simulink model "howard_lin_r2013a_20160128"  (R2013a)
settings: Solver=ode45  StartTime=0.0  StopTime=tFinal  RelTol=1e-3
PreLoadFcn:
  | OAT=30;
  | Temp=68;
  | 
  | Rn=29;
  | Rx=69;
  | Tn=180;
  | Tx=120;
  | 
  | Hc=114/86400;
  | Ha=1.61/86400;
  | %Hf=1.08/86400;
  | Hf=1.745/86400;
  | Ho=283/86400;
  | 
  | tau=40;
  | FILTER_DELAY = 5;
  | 
  | K2=1;
  | K3=1;
  | Ki=1e-5;
  | Kp=2;
  | Kd=800;
  | Kf=1;
  | compGain=400;  % gain in TCOMP of house control
  | Kei=Ki*2;
  | Kep=Kp*2;
  | 
  | % From match to thermo20160128.xlsx
  | sNoise=0.001;
  | SET = [0 60 18861 18862; 68 62 68 68]';
  | otherHeat=[0 1000 6000; .0002 .001 .0005]';
  | tFinal = 24132;
InitFcn:
  | Ta0=Temp;
  | Tw0 = (Temp*Ha + OAT*Ho)/(Ho+Ha);
  | Tb0=max(min(interp1([Rn Rx],[Tn Tx],OAT), Tn),Tx);
  | Tc0 = ((Ha+Hc)*Ta0 - Ha*Tw0) / Hc;
  | D0 =max(min( Hc*(Tc0-Ta0)/(Hf*(Tb0-Tc0)), 1), 1e-32);
settings Model: Creator=210023782  LastModifiedBy=210023782
settings DataIOCC: InitialState=xinHouse  LimitDataPoints=off  SaveState=on  StateSaveName=xoutHouse

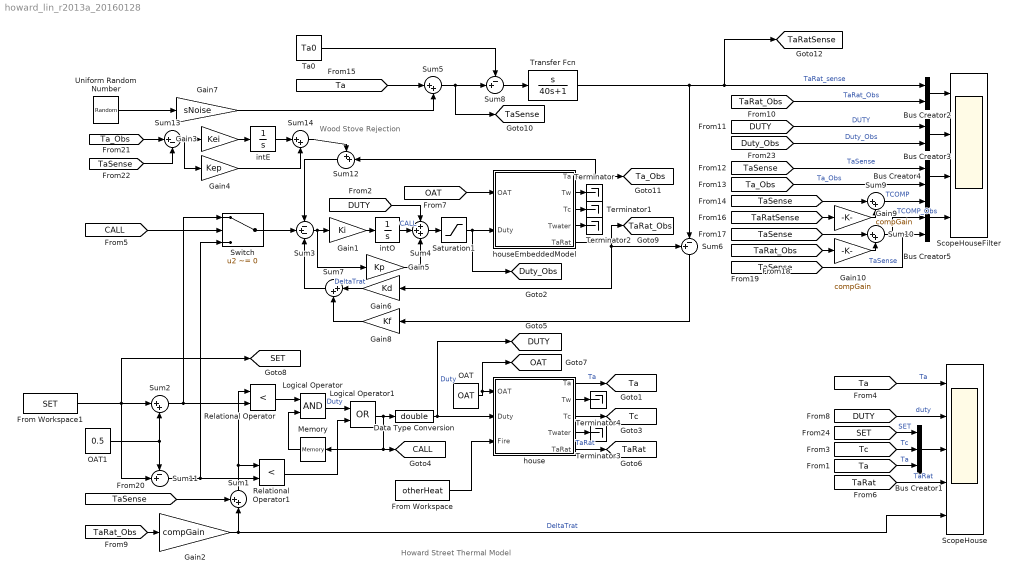
== system howard_lin_r2013a_20160128 ==
  note: Howard Street Thermal Model
  note: Wood Stove Rejection
  Bus Creator1 : BusCreator  Inputs=3
  Bus Creator2 : BusCreator  Inputs=2
  Bus Creator3 : BusCreator  Inputs=2
  Bus Creator4 : BusCreator  Inputs=2
  Bus Creator5 : BusCreator  Inputs=3
  Data Type Conversion : DataTypeConversion  OutDataTypeStr=double
  From Workspace : FromWorkspace  VariableName=otherHeat  SampleTime=1  OutputAfterFinalValue=Holding final value
  From Workspace1 : FromWorkspace  VariableName=SET  SampleTime=1  OutputAfterFinalValue=Holding final value
  Gain1 : Gain  Gain=Ki
  Gain10 : Gain  Gain=compGain
  Gain2 : Gain  Gain=compGain
  Gain3 : Gain  Gain=Kei
  Gain4 : Gain  Gain=Kep
  Gain5 : Gain  Gain=Kp
  Gain6 : Gain  Gain=Kd
  Gain7 : Gain  Gain=sNoise
  Gain8 : Gain  Gain=Kf
  Gain9 : Gain  Gain=compGain
  Logical Operator : Logic  AllPortsSameDT=off  OutDataTypeStr=boolean
  Logical Operator1 : Logic  Operator=OR  AllPortsSameDT=off  OutDataTypeStr=boolean
  Memory : Memory
  OAT : Constant  Value=OAT
  OAT1 : Constant  Value=0.5
  Relational Operator : RelationalOperator  Operator=<  OutDataTypeStr=boolean
  Relational Operator1 : RelationalOperator  Operator=<  OutDataTypeStr=boolean
  Saturation1 : Saturate  UpperLimit=1.0  LowerLimit=1e-32
  ScopeHouse : Scope  NumInputPorts=5
      settings: ShowLegends=on  YMin=-75~-40~-5~-5~-5  YMax=75~70~5~5~5  Decimation=2
  ScopeHouseFilter : Scope  NumInputPorts=4
      settings: ShowLegends=on  YMin=-75~-40~-10~-5  YMax=75~70~10~5  SaveName=ScopeData4  Decimation=2
  Sum1 : Sum  Inputs=++|
  Sum{2,5,7,9..10,14} (6 alike) : Sum  Inputs=|++
  Sum11 : Sum  Inputs=-+|
  Sum12 : Sum  Inputs=++|
  Sum13 : Sum  Inputs=|+-
  Sum3 : Sum  Inputs=-+-
  Sum4 : Sum  Inputs=+++
  Sum6 : Sum  Inputs=+-|
  Sum8 : Sum  Inputs=-+|
  Switch : Switch  Criteria=u2 ~= 0
  Ta0 : Constant  Value=Ta0
  Terminator{,1..4} (5 alike) : Terminator
  Transfer Fcn : TransferFcn  Numerator=[1 0]  Denominator=[40 1]
  Uniform Random Number : UniformRandomNumber  SampleTime=FILTER_DELAY
  house : Subsystem
  houseEmbeddedModel : Subsystem
  intE : Integrator  LimitOutput=on  UpperSaturationLimit=10  LowerSaturationLimit=-10
  intO : Integrator  LimitOutput=on  UpperSaturationLimit=1  LowerSaturationLimit=-1
  tag scope: CALL=global, DUTY=global, Duty_Obs=global, OAT=global, SET=global, Ta=global, TaRat=global, TaRatSense=global, TaRat_Obs=global, TaSense=global, Ta_Obs=global, Tc=global
  wires:
  OAT/1 -> [OAT], house/1(OAT)
  house/1(Ta) -> [Ta]  "Ta"
  house/2(Tw) -> Terminator4/1
  house/3(Tc) -> [Tc]
  house/4(Twater) -> Terminator3/1
  Bus Creator2/1 -> ScopeHouseFilter/1
  [Ta] -> ScopeHouse/1  "Ta"
  house/5(TaRat) -> [TaRat]  "TaRat"
  [TaRat] -> ScopeHouse/4  "TaRat"
  Logical Operator/1 -> Logical Operator1/1  "Duty"
  Gain2/1 -> ScopeHouse/5, Sum1/2  "DeltaTrat"
  [OAT] -> houseEmbeddedModel/1(OAT)
  houseEmbeddedModel/1(Ta) -> Sum12/2, [Ta_Obs]
  Sum3/1 -> Gain1/1, Gain5/1
  Sum4/1 -> Saturation1/1
  Gain1/1 -> intO/1
  Saturation1/1 -> houseEmbeddedModel/2(Duty), [Duty_Obs]
  [TaRat_Obs] -> Gain2/1
  houseEmbeddedModel/5(TaRat) -> Sum6/1, Gain6/1, [TaRat_Obs]
  houseEmbeddedModel/2(Tw) -> Terminator/1
  houseEmbeddedModel/3(Tc) -> Terminator1/1
  houseEmbeddedModel/4(Twater) -> Terminator2/1
  Uniform Random Number/1 -> Gain7/1
  Sum5/1 -> [TaSense], Sum8/2
  Transfer Fcn/1 -> [TaRatSense], Bus Creator2/1, Sum6/2  "TaRat_sense"
  Sum6/1 -> Gain8/1
  Sum7/1 -> Sum3/3
  Gain6/1 -> Sum7/1  "DeltaTrat"
  Gain8/1 -> Sum7/2
  [TaRat_Obs] -> Bus Creator2/2  "TaRat_Obs"
  [DUTY] -> Bus Creator3/1  "DUTY"
  Bus Creator3/1 -> ScopeHouseFilter/2
  [Ta] -> Sum5/1
  Gain7/1 -> Sum5/2
  Ta0/1 -> Sum8/1
  Sum8/1 -> Transfer Fcn/1
  [TaSense] -> Bus Creator4/1  "TaSense"
  [Ta_Obs] -> Bus Creator4/2  "Ta_Obs"
  Bus Creator4/1 -> ScopeHouseFilter/3
  Bus Creator5/1 -> ScopeHouseFilter/4
  [TaRatSense] -> Gain9/1
  [TaSense] -> Sum9/1
  Gain9/1 -> Sum9/2
  Sum9/1 -> Bus Creator5/1  "TCOMP"
  [TaRat_Obs] -> Gain10/1
  [TaSense] -> Sum10/1
  Gain10/1 -> Sum10/2
  Sum10/1 -> Bus Creator5/2  "TCOMP_Obs"
  [TaSense] -> Bus Creator5/3  "TaSense"
  Sum1/1 -> Relational Operator1/1, Relational Operator/1
  OAT1/1 -> Sum11/1, Sum2/2
  Sum2/1 -> Switch/1, Relational Operator/2
  Relational Operator/1 -> Logical Operator/1
  [TaSense] -> Sum1/1
  Data Type Conversion/1 -> house/2(Duty), [DUTY]  "Duty"
  Memory/1 -> Logical Operator/2
  Relational Operator1/1 -> Logical Operator1/2
  Sum11/1 -> Relational Operator1/2, Switch/3
  intO/1 -> Sum4/2  "CALL"
  Gain5/1 -> Sum4/3
  [DUTY] -> Sum4/1
  Switch/1 -> Sum3/2
  [CALL] -> Switch/2
  From Workspace/1 -> house/3(Fire)
  Sum12/1 -> Sum3/1
  [Ta_Obs] -> Sum13/1
  [TaSense] -> Sum13/2
  Sum13/1 -> Gain4/1, Gain3/1
  Gain3/1 -> intE/1
  intE/1 -> Sum14/1
  Gain4/1 -> Sum14/2
  Sum14/1 -> Sum12/1
  [Duty_Obs] -> Bus Creator3/2  "Duty_Obs"
  Logical Operator1/1 -> Memory/1, [CALL], Data Type Conversion/1
  [DUTY] -> ScopeHouse/2  "duty"
  From Workspace1/1 -> [SET], Sum11/2, Sum2/1
  [Ta] -> Bus Creator1/3  "Ta"
  [Tc] -> Bus Creator1/2  "Tc"
  [SET] -> Bus Creator1/1  "SET"
  Bus Creator1/1 -> ScopeHouse/3

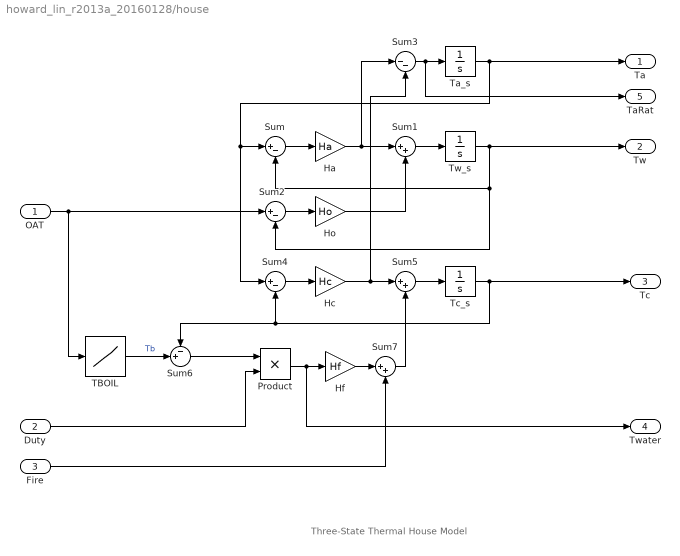
== system howard_lin_r2013a_20160128/house ==
  note: Three-State Thermal House Model
  OAT : Inport
  Duty : Inport  Port=2
  Fire : Inport  Port=3
  Ha : Gain  Gain=Ha
  Hc : Gain  Gain=Hc
  Hf : Gain  Gain=Hf
  Ho : Gain  Gain=Ho
  Product : Product
  Sum : Sum  Inputs=|+-
  Sum1 : Sum  Inputs=|++
  Sum2 : Sum  Inputs=|+-
  Sum3 : Sum  Inputs=|--
  Sum4 : Sum  Inputs=|+-
  Sum5 : Sum  Inputs=|++
  Sum6 : Sum  Inputs=-+|
  Sum7 : Sum  Inputs=|++
  TBOIL : Lookup_n-D  NumberOfTableDimensions=1  BreakpointsForDimension1=[Rn Rx]  Table=[Tn Tx]  ExtrapMethod=Clip  RndMeth=Simplest  InputSameDT=on
  Ta_s : Integrator  InitialCondition=Ta0
  Tc_s : Integrator  InitialCondition=Tc0
  Tw_s : Integrator  InitialCondition=Tw0
  Ta : Outport
  Tw : Outport  Port=2
  Tc : Outport  Port=3
  Twater : Outport  Port=4
  TaRat : Outport  Port=5
  wires:
  Ta_s/1 -> Ta/1, Sum4/1, Sum/1
  Sum/1 -> Ha/1
  Sum2/1 -> Ho/1
  Tw_s/1 -> Tw/1, Sum/2, Sum2/2
  Ha/1 -> Sum3/1, Sum1/1
  Sum4/1 -> Hc/1
  Ho/1 -> Sum1/2
  Sum1/1 -> Tw_s/1
  Sum3/1 -> TaRat/1, Ta_s/1
  Sum5/1 -> Tc_s/1
  Tc_s/1 -> Tc/1, Sum6/1, Sum4/2
  Hc/1 -> Sum3/2, Sum5/1
  Product/1 -> Twater/1, Hf/1
  Duty/1 -> Product/2
  Sum6/1 -> Product/1
  TBOIL/1 -> Sum6/2  "Tb"
  Hf/1 -> Sum7/1
  Sum7/1 -> Sum5/2
  Fire/1 -> Sum7/2
  OAT/1 -> TBOIL/1, Sum2/1

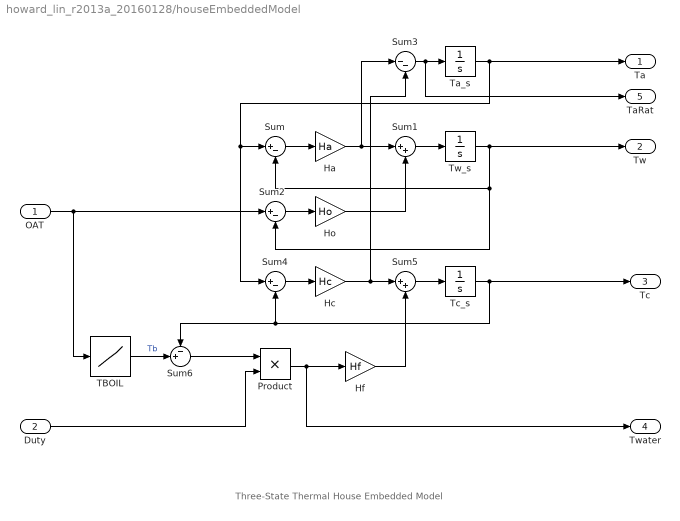
== system howard_lin_r2013a_20160128/houseEmbeddedModel ==
  note: Three-State Thermal House Embedded Model
  OAT : Inport
  Duty : Inport  Port=2
  Ha : Gain  Gain=Ha
  Hc : Gain  Gain=Hc
  Hf : Gain  Gain=Hf
  Ho : Gain  Gain=Ho
  Product : Product
  Sum : Sum  Inputs=|+-
  Sum1 : Sum  Inputs=|++
  Sum2 : Sum  Inputs=|+-
  Sum3 : Sum  Inputs=|--
  Sum4 : Sum  Inputs=|+-
  Sum5 : Sum  Inputs=|++
  Sum6 : Sum  Inputs=-+|
  TBOIL : Lookup_n-D  NumberOfTableDimensions=1  BreakpointsForDimension1=[Rn Rx]  Table=[Tn Tx]  ExtrapMethod=Clip  RndMeth=Simplest  InputSameDT=on
  Ta_s : Integrator  InitialCondition=Ta0
  Tc_s : Integrator  InitialCondition=Tc0
  Tw_s : Integrator  InitialCondition=Tw0
  Ta : Outport
  Tw : Outport  Port=2
  Tc : Outport  Port=3
  Twater : Outport  Port=4
  TaRat : Outport  Port=5
  wires:
  Sum6/1 -> Product/1
  Hf/1 -> Sum5/2
  Duty/1 -> Product/2
  Product/1 -> Hf/1, Twater/1
  Hc/1 -> Sum5/1, Sum3/2
  Tc_s/1 -> Sum4/2, Sum6/1, Tc/1
  Sum5/1 -> Tc_s/1
  Sum3/1 -> Ta_s/1, TaRat/1
  Sum1/1 -> Tw_s/1
  Ho/1 -> Sum1/2
  Sum4/1 -> Hc/1
  Ha/1 -> Sum1/1, Sum3/1
  Tw_s/1 -> Sum2/2, Sum/2, Tw/1
  Sum2/1 -> Ho/1
  Sum/1 -> Ha/1
  Ta_s/1 -> Sum/1, Sum4/1, Ta/1
  TBOIL/1 -> Sum6/2  "Tb"
  OAT/1 -> TBOIL/1, Sum2/1
